simulink model "ROI"  (R2017a)
settings: Solver=FixedStepAuto  StartTime=0.0  StopTime=10.0  FixedStep=1/5  RelTol=1e-3
settings Model: Creator=ChiChaChai  LastModifiedBy=ChiChaChai

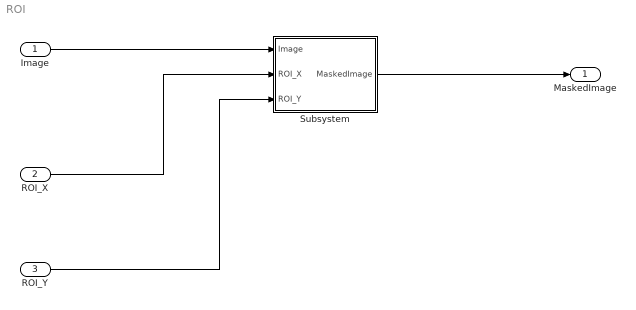
== system ROI ==
  Image : Inport
  ROI_X : Inport  Port=2
  ROI_Y : Inport  Port=3
  Subsystem : Subsystem
  "MaskedImage " : Outport
  wires:
  Image/1 -> Subsystem/1(Image)
  ROI_X/1 -> Subsystem/2(ROI_X)
  ROI_Y/1 -> Subsystem/3(ROI_Y)
  Subsystem/1("MaskedImage ") -> "MaskedImage "/1

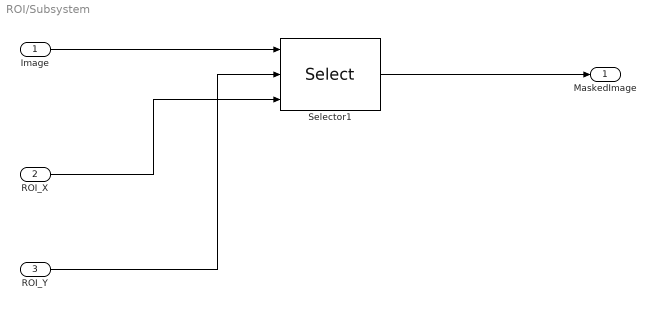
== system ROI/Subsystem ==
  Image : Inport
  ROI_X : Inport  Port=2
  ROI_Y : Inport  Port=3
  Selector1 : Selector  NumberOfDimensions=2  InputPortWidth=3  IndexOptions=Index vector (port),Index vector (port)  Indices=[20:280],[80:150]  OutputSizes=1,1
  "MaskedImage " : Outport
  wires:
  Image/1 -> Selector1/1
  Selector1/1 -> "MaskedImage "/1
  ROI_X/1 -> Selector1/3
  ROI_Y/1 -> Selector1/2
